simulink model "Roadsense_ScenarioSensorSource"  (R2025b)
settings: Solver=FixedStepDiscrete  StartTime=0.0  StopTime=25  FixedStep=RsTsBase  RelTol=1e-3
undefined symbols (not defined in the file or in its folder): RsMaxLidarPoints, RsTsScenario
settings Model: DataDictionary=Roadsense_Data.sldd  Creator=ragur  LastModifiedBy=ragur

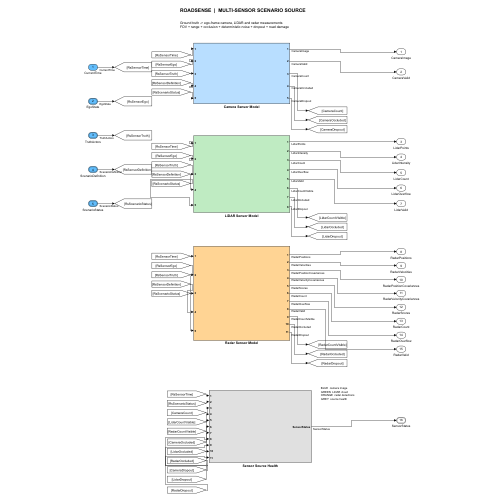
[thumbnail: Simulink's stored preview of the top-level diagram]
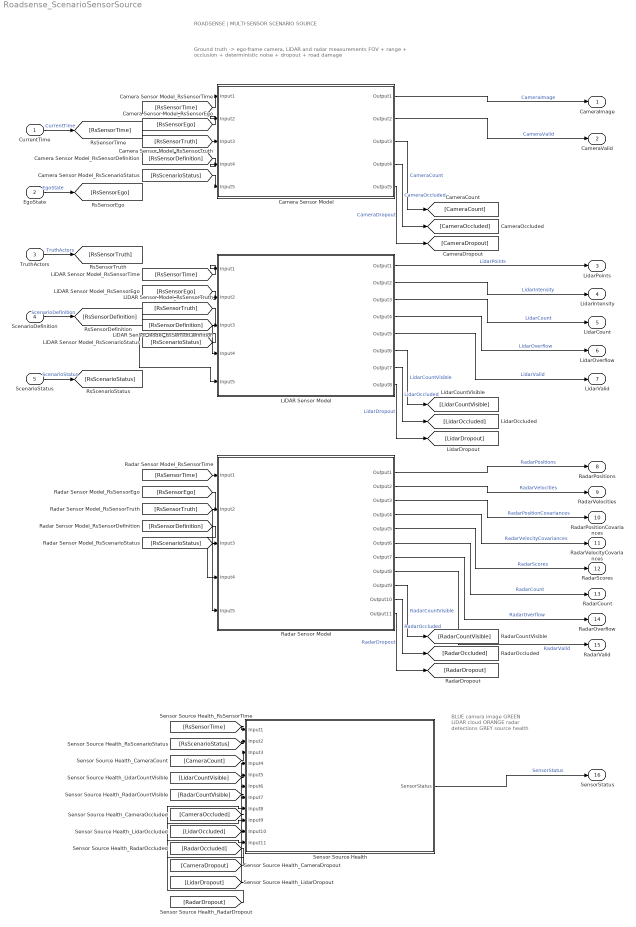
== system Roadsense_ScenarioSensorSource ==
  note: ROADSENSE | MULTI-SENSOR SCENARIO SOURCE
  note: Ground truth -> ego-frame camera, LiDAR and radar measurements
      | FOV + range + occlusion + deterministic noise + dropout + road damage
  note: BLUE  camera image
      | GREEN  LiDAR cloud
      | ORANGE  radar detections
      | GREY  source health
  CurrentTime : Inport  OutDataTypeStr=double  SampleTime=RsTsScenario
  EgoState : Inport  Port=2  OutDataTypeStr=Bus: RsEgoStateBus  SampleTime=RsTsScenario
  TruthActors : Inport  Port=3  OutDataTypeStr=Bus: RsScenarioActorListBus  SampleTime=RsTsScenario
  ScenarioDefinition : Inport  Port=4  OutDataTypeStr=Bus: RsScenarioDefinitionBus  SampleTime=RsTsScenario
  ScenarioStatus : Inport  Port=5  OutDataTypeStr=Bus: RsScenarioStatusBus  SampleTime=RsTsScenario
  Camera Sensor Model : Subsystem
  LiDAR Sensor Model : Subsystem
  Radar Sensor Model : Subsystem
  Sensor Source Health : Subsystem
  CameraImage : Outport  OutDataTypeStr=uint8  PortDimensions=[480 640 3]
  CameraValid : Outport  Port=2  OutDataTypeStr=boolean  PortDimensions=1
  LidarPoints : Outport  Port=3  OutDataTypeStr=single  PortDimensions=[120000 3]
  LidarIntensity : Outport  Port=4  OutDataTypeStr=single  PortDimensions=[120000 1]
  LidarCount : Outport  Port=5  OutDataTypeStr=uint32  PortDimensions=1
  LidarOverflow : Outport  Port=6  OutDataTypeStr=boolean  PortDimensions=1
  LidarValid : Outport  Port=7  OutDataTypeStr=boolean  PortDimensions=1
  RadarPositions : Outport  Port=8  OutDataTypeStr=single  PortDimensions=[256 3]
  RadarVelocities : Outport  Port=9  OutDataTypeStr=single  PortDimensions=[256 3]
  RadarPositionCovariances : Outport  Port=10  OutDataTypeStr=single  PortDimensions=[3 3 256]
  RadarVelocityCovariances : Outport  Port=11  OutDataTypeStr=single  PortDimensions=[3 3 256]
  RadarScores : Outport  Port=12  OutDataTypeStr=single  PortDimensions=[256 1]
  RadarCount : Outport  Port=13  OutDataTypeStr=uint16  PortDimensions=1
  RadarOverflow : Outport  Port=14  OutDataTypeStr=boolean  PortDimensions=1
  RadarValid : Outport  Port=15  OutDataTypeStr=boolean  PortDimensions=1
  SensorStatus : Outport  Port=16  OutDataTypeStr=Bus: RsScenarioSensorStatusBus
  wires:
  CurrentTime/1 -> [RsSensorTime]  "CurrentTime"
  EgoState/1 -> [RsSensorEgo]  "EgoState"
  TruthActors/1 -> [RsSensorTruth]  "TruthActors"
  ScenarioDefinition/1 -> [RsSensorDefinition]  "ScenarioDefinition"
  ScenarioStatus/1 -> [RsScenarioStatus]  "ScenarioStatus"
  [RsSensorTime] -> Camera Sensor Model/1(Input1)
  [RsSensorEgo] -> Camera Sensor Model/2(Input2)
  [RsSensorTruth] -> Camera Sensor Model/3(Input3)
  [RsSensorDefinition] -> Camera Sensor Model/4(Input4)
  [RsScenarioStatus] -> Camera Sensor Model/5(Input5)
  [RsSensorTime] -> LiDAR Sensor Model/1(Input1)
  [RsSensorEgo] -> LiDAR Sensor Model/2(Input2)
  [RsSensorTruth] -> LiDAR Sensor Model/3(Input3)
  [RsSensorDefinition] -> LiDAR Sensor Model/4(Input4)
  [RsScenarioStatus] -> LiDAR Sensor Model/5(Input5)
  [RsSensorTime] -> Radar Sensor Model/1(Input1)
  [RsSensorEgo] -> Radar Sensor Model/2(Input2)
  [RsSensorTruth] -> Radar Sensor Model/3(Input3)
  [RsSensorDefinition] -> Radar Sensor Model/4(Input4)
  [RsScenarioStatus] -> Radar Sensor Model/5(Input5)
  Camera Sensor Model/1(Output1) -> CameraImage/1  "CameraImage"
  Camera Sensor Model/2(Output2) -> CameraValid/1  "CameraValid"
  LiDAR Sensor Model/1(Output1) -> LidarPoints/1  "LidarPoints"
  LiDAR Sensor Model/2(Output2) -> LidarIntensity/1  "LidarIntensity"
  LiDAR Sensor Model/3(Output3) -> LidarCount/1  "LidarCount"
  LiDAR Sensor Model/4(Output4) -> LidarOverflow/1  "LidarOverflow"
  LiDAR Sensor Model/5(Output5) -> LidarValid/1  "LidarValid"
  Radar Sensor Model/1(Output1) -> RadarPositions/1  "RadarPositions"
  Radar Sensor Model/2(Output2) -> RadarVelocities/1  "RadarVelocities"
  Radar Sensor Model/3(Output3) -> RadarPositionCovariances/1  "RadarPositionCovariances"
  Radar Sensor Model/4(Output4) -> RadarVelocityCovariances/1  "RadarVelocityCovariances"
  Radar Sensor Model/5(Output5) -> RadarScores/1  "RadarScores"
  Radar Sensor Model/6(Output6) -> RadarCount/1  "RadarCount"
  Radar Sensor Model/7(Output7) -> RadarOverflow/1  "RadarOverflow"
  Radar Sensor Model/8(Output8) -> RadarValid/1  "RadarValid"
  Camera Sensor Model/3(Output3) -> [CameraCount]  "CameraCount"
  Camera Sensor Model/4(Output4) -> [CameraOccluded]  "CameraOccluded"
  Camera Sensor Model/5(Output5) -> [CameraDropout]  "CameraDropout"
  LiDAR Sensor Model/6(Output6) -> [LidarCountVisible]  "LidarCountVisible"
  LiDAR Sensor Model/7(Output7) -> [LidarOccluded]  "LidarOccluded"
  LiDAR Sensor Model/8(Output8) -> [LidarDropout]  "LidarDropout"
  Radar Sensor Model/9(Output9) -> [RadarCountVisible]  "RadarCountVisible"
  Radar Sensor Model/10(Output10) -> [RadarOccluded]  "RadarOccluded"
  Radar Sensor Model/11(Output11) -> [RadarDropout]  "RadarDropout"
  [RsSensorTime] -> Sensor Source Health/1(Input1)
  [RsScenarioStatus] -> Sensor Source Health/2(Input2)
  [CameraCount] -> Sensor Source Health/3(Input3)
  [LidarCountVisible] -> Sensor Source Health/4(Input4)
  [RadarCountVisible] -> Sensor Source Health/5(Input5)
  [CameraOccluded] -> Sensor Source Health/6(Input6)
  [LidarOccluded] -> Sensor Source Health/7(Input7)
  [RadarOccluded] -> Sensor Source Health/8(Input8)
  [CameraDropout] -> Sensor Source Health/9(Input9)
  [LidarDropout] -> Sensor Source Health/10(Input10)
  [RadarDropout] -> Sensor Source Health/11(Input11)
  Sensor Source Health/1(SensorStatus) -> SensorStatus/1  "SensorStatus"

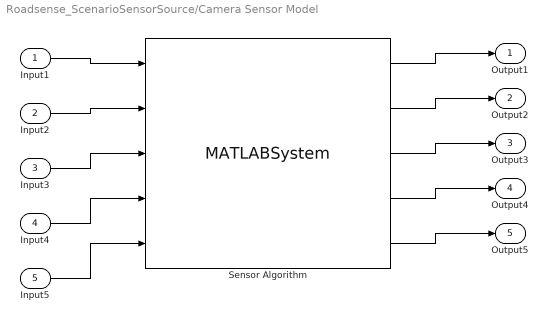
== system Roadsense_ScenarioSensorSource/Camera Sensor Model ==
  Input1 : Inport
  Input2 : Inport  Port=2
  Input3 : Inport  Port=3
  Input4 : Inport  Port=4
  Input5 : Inport  Port=5
  Sensor Algorithm : MATLABSystem  System=RoadsenseScenarioCameraSystem  HorizontalFOV=RsScenarioCameraHorizontalFOV  MaximumRange=RsScenarioCameraRange  FocalLength=RsCameraFocalLength  PrincipalPoint=RsCameraPrincipalPoint  CameraHeight=RsCameraHeight  PitchDown=RsCameraPitchDown  SimulateUsing=Interpreted execution
      mask Type: RoadsenseScenarioCameraSystem
  Output1 : Outport
  Output2 : Outport  Port=2
  Output3 : Outport  Port=3
  Output4 : Outport  Port=4
  Output5 : Outport  Port=5
  wires:
  Input1/1 -> Sensor Algorithm/1
  Input2/1 -> Sensor Algorithm/2
  Input3/1 -> Sensor Algorithm/3
  Input4/1 -> Sensor Algorithm/4
  Input5/1 -> Sensor Algorithm/5
  Sensor Algorithm/1 -> Output1/1
  Sensor Algorithm/2 -> Output2/1
  Sensor Algorithm/3 -> Output3/1
  Sensor Algorithm/4 -> Output4/1
  Sensor Algorithm/5 -> Output5/1

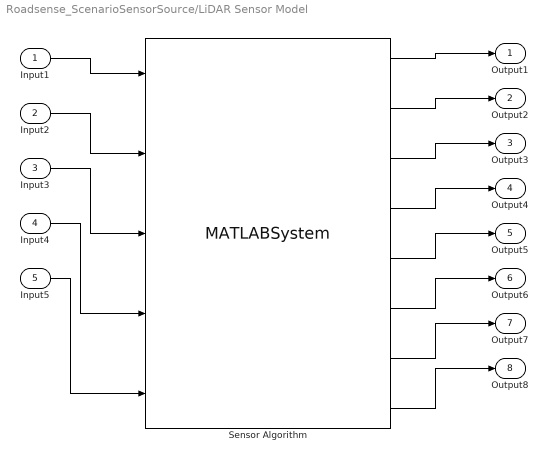
== system Roadsense_ScenarioSensorSource/LiDAR Sensor Model ==
  Input1 : Inport
  Input2 : Inport  Port=2
  Input3 : Inport  Port=3
  Input4 : Inport  Port=4
  Input5 : Inport  Port=5
  Sensor Algorithm : MATLABSystem  System=RoadsenseScenarioLidarSystem  MaximumRange=RsScenarioLidarRange  MaximumPoints=double(RsMaxLidarPoints)  SimulateUsing=Interpreted execution
      mask Type: RoadsenseScenarioLidarSystem
  Output1 : Outport
  Output2 : Outport  Port=2
  Output3 : Outport  Port=3
  Output4 : Outport  Port=4
  Output5 : Outport  Port=5
  Output6 : Outport  Port=6
  Output7 : Outport  Port=7
  Output8 : Outport  Port=8
  wires:
  Input1/1 -> Sensor Algorithm/1
  Input2/1 -> Sensor Algorithm/2
  Input3/1 -> Sensor Algorithm/3
  Input4/1 -> Sensor Algorithm/4
  Input5/1 -> Sensor Algorithm/5
  Sensor Algorithm/1 -> Output1/1
  Sensor Algorithm/2 -> Output2/1
  Sensor Algorithm/3 -> Output3/1
  Sensor Algorithm/4 -> Output4/1
  Sensor Algorithm/5 -> Output5/1
  Sensor Algorithm/6 -> Output6/1
  Sensor Algorithm/7 -> Output7/1
  Sensor Algorithm/8 -> Output8/1

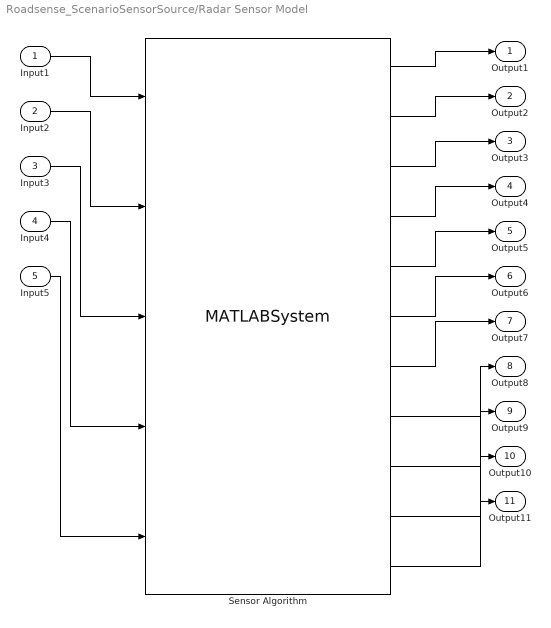
== system Roadsense_ScenarioSensorSource/Radar Sensor Model ==
  Input1 : Inport
  Input2 : Inport  Port=2
  Input3 : Inport  Port=3
  Input4 : Inport  Port=4
  Input5 : Inport  Port=5
  Sensor Algorithm : MATLABSystem  System=RoadsenseScenarioRadarSystem  MaximumRange=RsScenarioRadarRange  HorizontalFOV=single(2.4434609413147)  PositionSigma=RsScenarioRadarPositionSigma  VelocitySigma=RsScenarioRadarVelocitySigma  SimulateUsing=Interpreted execution
      mask Type: RoadsenseScenarioRadarSystem
  Output1 : Outport
  Output2 : Outport  Port=2
  Output3 : Outport  Port=3
  Output4 : Outport  Port=4
  Output5 : Outport  Port=5
  Output6 : Outport  Port=6
  Output7 : Outport  Port=7
  Output8 : Outport  Port=8
  Output9 : Outport  Port=9
  Output10 : Outport  Port=10
  Output11 : Outport  Port=11
  wires:
  Input1/1 -> Sensor Algorithm/1
  Input2/1 -> Sensor Algorithm/2
  Input3/1 -> Sensor Algorithm/3
  Input4/1 -> Sensor Algorithm/4
  Input5/1 -> Sensor Algorithm/5
  Sensor Algorithm/1 -> Output1/1
  Sensor Algorithm/2 -> Output2/1
  Sensor Algorithm/3 -> Output3/1
  Sensor Algorithm/4 -> Output4/1
  Sensor Algorithm/5 -> Output5/1
  Sensor Algorithm/6 -> Output6/1
  Sensor Algorithm/7 -> Output7/1
  Sensor Algorithm/8 -> Output8/1
  Sensor Algorithm/9 -> Output9/1
  Sensor Algorithm/10 -> Output10/1
  Sensor Algorithm/11 -> Output11/1

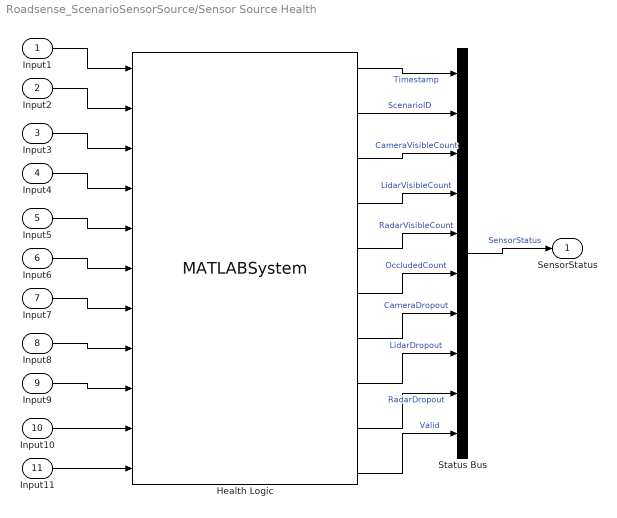
== system Roadsense_ScenarioSensorSource/Sensor Source Health ==
  Input1 : Inport
  Input2 : Inport  Port=2
  Input3 : Inport  Port=3
  Input4 : Inport  Port=4
  Input5 : Inport  Port=5
  Input6 : Inport  Port=6
  Input7 : Inport  Port=7
  Input8 : Inport  Port=8
  Input9 : Inport  Port=9
  Input10 : Inport  Port=10
  Input11 : Inport  Port=11
  Health Logic : MATLABSystem  System=RoadsenseScenarioSensorStatusSystem  SimulateUsing=Interpreted execution
      mask Type: RoadsenseScenarioSensorStatusSystem
  Status Bus : BusCreator  Inputs=10  OutDataTypeStr=Bus: RsScenarioSensorStatusBus
  SensorStatus : Outport  OutDataTypeStr=Bus: RsScenarioSensorStatusBus
  wires:
  Input1/1 -> Health Logic/1
  Input2/1 -> Health Logic/2
  Input3/1 -> Health Logic/3
  Input4/1 -> Health Logic/4
  Input5/1 -> Health Logic/5
  Input6/1 -> Health Logic/6
  Input7/1 -> Health Logic/7
  Input8/1 -> Health Logic/8
  Input9/1 -> Health Logic/9
  Input10/1 -> Health Logic/10
  Input11/1 -> Health Logic/11
  Health Logic/1 -> Status Bus/1  "Timestamp"
  Health Logic/2 -> Status Bus/2  "ScenarioID"
  Health Logic/3 -> Status Bus/3  "CameraVisibleCount"
  Health Logic/4 -> Status Bus/4  "LidarVisibleCount"
  Health Logic/5 -> Status Bus/5  "RadarVisibleCount"
  Health Logic/6 -> Status Bus/6  "OccludedCount"
  Health Logic/7 -> Status Bus/7  "CameraDropout"
  Health Logic/8 -> Status Bus/8  "LidarDropout"
  Health Logic/9 -> Status Bus/9  "RadarDropout"
  Health Logic/10 -> Status Bus/10  "Valid"
  Status Bus/1 -> SensorStatus/1  "SensorStatus"
